simulink model "twelve_oclock"  (Simulink 6.6)
settings: Solver=FixedStepDiscrete  StartTime=0.0  StopTime=10.0  FixedStep=1  RelTol=1e-3
settings Model: Creator=vBuskirk  LastModifiedBy=vBuskirk

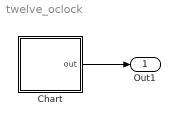
== system twelve_oclock ==
  Chart : Stateflow chart
  Out1 : Outport
  wires:
  Chart/1(out) -> Out1/1

== stateflow chart Chart ==
  state s10000
  state s11000
  state s12000
  state s11100
  state s11200
  state s12100
  state s12200
  state s12120
  state s12110
  state s12210
  state s12220
  state s11121
  state s11110
  state s11120
  state s11220
  state s11210
  state s11122
  state s11111
  state s11112
  state s11211
  state s11212
  state s11221
  state s11222
  state s12111
  state s12112
  state s12121
  state s12122
  state s12211
  state s12212
  state s12221
  state s12222
  (default) -> s10000
  s10000 -> s11000 [order 2]
  s10000 -> s12000 [order 1]
  s11000 -> s11100 [order 1]
  s11000 -> s11200 [order 2]
  s12000 -> s12100 [order 1]
  s12000 -> s12200 [order 2]
  s12200 -> s12210 [order 1]
  s12200 -> s12220 [order 2]
  s12100 -> s12110 [order 2]
  s12100 -> s12120 [order 1]
  s11100 -> s11110 [order 1]
  s11100 -> s11120 [order 2]
  s11110 -> s11111 [order 1] : / out=11111;
  s11110 -> s11112 [order 2] : / out=11112;
  s11120 -> s11121 [order 1] : / out=11121;
  s11120 -> s11122 [order 2] : / out=11122;
  s11210 -> s11211 [order 1] : / out=11211;
  s11210 -> s11212 [order 2] : / out=11212;
  s11220 -> s11221 [order 1] : / out=11221;
  s11220 -> s11222 [order 2] : / out=11222;
  s11200 -> s11210 [order 1]
  s11200 -> s11220 [order 2]
  s12110 -> s12111 [order 1] : / out=12111;
  s12110 -> s12112 [order 2] : / out=12112;
  s12120 -> s12121 [order 2] : / out=12121;
  s12120 -> s12122 [order 1] : / out=12122;
  s12210 -> s12211 [order 1] : / out=12211;
  s12210 -> s12212 [order 2] : / out=12212;
  s12220 -> s12221 [order 1] : / out=12221;
  s12220 -> s12222 [order 2] : / out=12222;
  data: out output double =-1
